simulink model "RadarSimulinkProjectRev011"  (R2024a)
settings: Solver=VariableStepAuto  StartTime=0.0  StopTime=0.0125*2  RelTol=1e-3
values from neighbouring files (symbols this model uses):
  AngleTime = SweepTime/10    (= 10000)    [InitializationOfVariablesRev000.m]    (also in InitializationOfVariablesRev001.m; InitializationOfVariablesRev002.m = 2000; InitializationOfVariablesRev003.m = 20000; InitializationOfVariablesRev004.m = 2097152)
  ASR_LUT = Rsamp    [InitializationOfVariablesRev003.m]    (also in InitializationOfVariablesRev004.m = round((R*2*SystemFs)/c); InitializationOfVariablesRev005.m = round((R*2*SystemFs)/c))
  Btn_Debounce = 20000    [InitializationOfVariablesRev003.m]    (also in InitializationOfVariablesRev004.m; InitializationOfVariablesRev005.m)
  ChirpNc = 128    [InitializationOfVariablesRev004.m]    (also in InitializationOfVariablesRev005.m)
  ChirpSizeLength = length(FCW)    [InitializationOfVariablesRev004.m]    (also in InitializationOfVariablesRev005.m = 16384)
  DeciFactor = 8    [InitializationOfVariablesRev005.m]
  FCW = [FCW_p1, FCW_p2]    [InitializationOfVariablesRev002.m]    (also in InitializationOfVariablesRev003.m; InitializationOfVariablesRev004.m = interp1(1:length(FCW_base), FCW_base,      linspace(1, lengt; InitializationOfVariablesRev005.m = f / SystemFs)
  RXFFTLength = 4096    [InitializationOfVariablesRev003.m]    (also in InitializationOfVariablesRev004.m = 1024; InitializationOfVariablesRev005.m = 2048)
  SweepTime = 100000    [InitializationOfVariablesRev000.m]    (also in InitializationOfVariablesRev001.m; InitializationOfVariablesRev002.m = 20000; InitializationOfVariablesRev003.m = 200000; InitializationOfVariablesRev004.m = 23068672)
undefined symbols (not defined in the file or in its folder): SignalGenerationForAnalysis, Subsystem, xc7a200tfbg676
libraries: hdlBasic x453, hdlUtilities x11, hdlDSPIP x11, vmcUtilities x1
(part 1 of 5)
settings Model: Creator=Cube II  LastModifiedBy=Cube II
settings ModelReferenceCC: UpdateModelReferenceTargets=IfOutOfDate

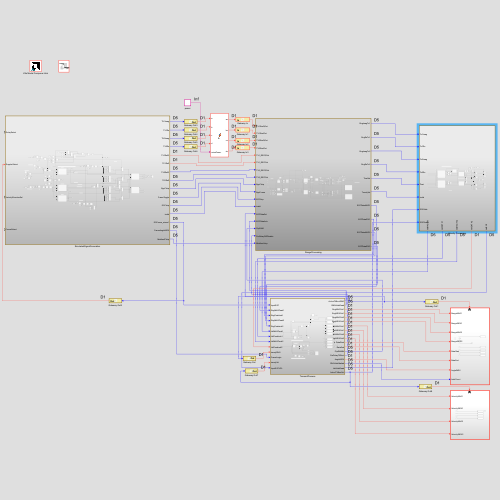
[thumbnail: Simulink's stored preview of the top-level diagram]
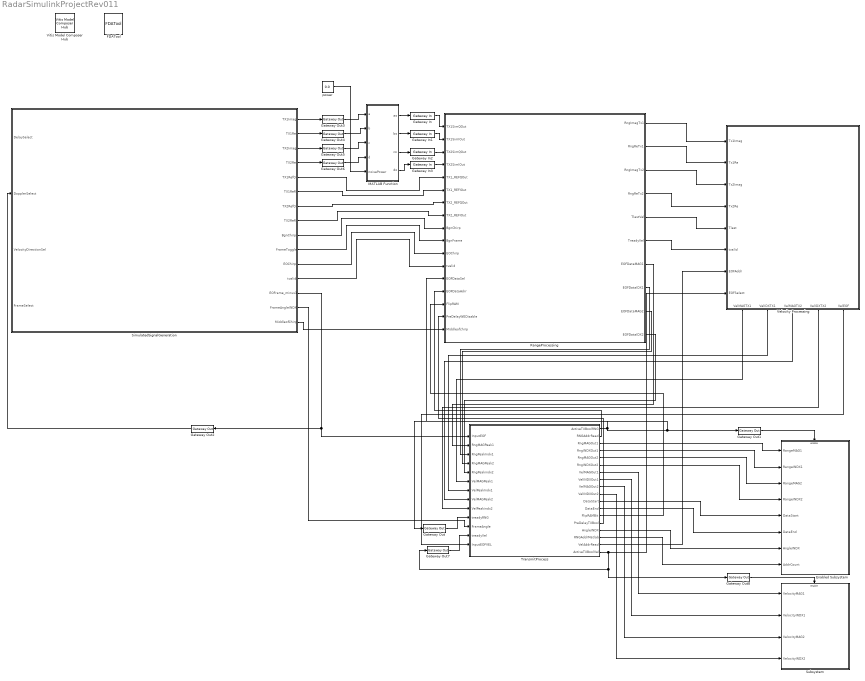
== system RadarSimulinkProjectRev011 ==
  Enabled Subsystem : Subsystem  TreatAsAtomicUnit=on
  FDATool : hdlUtilities/FDATool  block_type=fdatool
      settings: infoedit=FDATool
  Gateway In{,1..3} (4 alike) : hdlBasic/Gateway In  gui_display_data_type=Fixed-point  arith_type=Signed (2's comp)  n_bits=16  bin_pt=14  preci_type=Single  exp_width=8  frac_width=24  rows=1  columns=1  quantization="Round  (unbiased: +/- Inf)"  overflow=Saturate  period=P1  UseAsADC=off  ADCChannel='1'  interface=None  automatic_assignment=on  address_offset=hex2dec('00')  intf_name=''  intf_description=''  default_value=0  timing_constraint=None  locs_specified=off  LOCs={}  io_standard={}  inherit_from_input=off  hdl_port=on  XmcBlockStatus=1  maskContainerNames=group4  block_type=gatewayin  block_config=sysgen:gateway_in_config  block_width_w=590  block_height_w=620  block_width=640  block_height=850
  Gateway Out{,1..8} (9 alike) : hdlBasic/Gateway Out  inherit_from_input=off  bool_to_boolean=off  hdl_port=on  rows=1  columns=1  UseAsDAC=off  DACChannel='1'  interface=None  automatic_assignment=on  address_offset=hex2dec('00')  intf_name=''  intf_description=''  timing_constraint=None  locs_specified=off  LOCs={}  io_standard={}  XmcBlockStatus=1  maskContainerNames=group4  block_type=gatewayout  block_config=sysgen:gateway_out_config  block_width_w=590  block_height_w=620  block_width=620  block_height=750
  MATLAB Function : MATLAB Function  TreatAsAtomicUnit=on
  RangeProcessing : Subsystem
  SimulatedSignalGeneration : Subsystem  SystemSampleTime=1/200e6
  Subsystem : Subsystem
  TransmitProcess : Subsystem
  Velocity Processing : Subsystem
      settings: PortSchema="{\"entries\":[{\"content\":{\"sides\":[{\"content\":{\"connectorIds\":[\"In1\",\"In2\",\"In3\",\"In4\",\"In5\",\"In6\",\"In7\",\"In8\"]},\"type\":\"ConnectorPlacement.EquallySpacedRectSide\",\"uuid\":\"28660edc-4300-4d13-b5c7-cb230341ceef\"},{\"content\":{\"side\":\"RIGHT\"},\"type\":\"ConnectorPlacement.EquallySpacedRectSide\",\"uuid\":\"0aea0b64-dbd9-49d9-980c-6712e9fa4544\"},{\"content\":{\"side\":\"TOP\"},\"type\":\"ConnectorPlacement.EquallySpacedRectSide\",\"uuid\":\"4015706e-c6eb-4ca9-b4bb-31c510b09214\"},{\"content\":{\"connectorIds\":[\"Out1\",\"Out2\",\"Out3\",\"Out4\",\"Out5\"],\"side\":\"BOTTOM\"},\"type\":\"ConnectorPlacement.EquallySpacedRectSide\",\"uuid\":\"e3ca7ed1-345c-4783-9732-f7a0ff2c5995\"}]},\"type\":\"ConnectorPlacement.EquallySpacedConnector\",\"uuid\":\"ab051aed-e004-4640-a7d2-fe89028938d7\"}],\"packageUris\":[\"http://schema.mathworks.com/mf0/Connector/R2020b\"],\"version\":\"1.0\"}"
  Vitis Model Composer Hub : vmcUtilities/Vitis Model Composer Hub  Tag=genX  CodeGeneration=off  SubsystemName=RangeProcessing  BlockHierPath=SignalGenerationForAnalysis/Subsystem  CompilationType=HDLCompilation  SubsystemType=HDLNode  ExportTypeV2=IP Catalog  StartColumn=1  NumberOfColumns=1  TargetDirectory=./netlist  exportDesign=off  analyzeDesign=on  validateDesignOnHw=off  ExportType=AI Engines  IpVendor=xilinx.com  IpLibrary=hls  IpVersion=1.0  IpHWLanguage=Verilog  AieCompilerOptions={}  AieSimulatorOptions={}  CreateTestbench=on  TestbenchStackSize=10  RunRtlSim=off  RunCSim=off  RunAieSim=off  AieSimTimeout=50000  RunAieSimProfiling=off  LaunchVitisAnalyzer=off  PlotOutput=off  RunX86Sim=off  X86SimTimeout=10  GenHwImage=off  GenLibadfXo=on  GenHwValidationCode=off  PlatformType=Not Specified  HwSystemType=Baremetal  HwValidationTarget=hw  ProjDevice=Artix-7 AC701 Evaluation Platform (xc7a200tfbg676-2)  ProjDevicePart=xc7a200tfbg676-2  AIEType=None  SamplePeriod=-1  ClockFrequency=200  DataPathParallelism=1  xilinxfamily=artix7  part=xc7a200t  speed=-2  package=fbg676  directory=./netlist\ip\RangeProcessing\src  testbench=off  incr_netlist=off  synthesis_tool=Vivado  clock_wrapper=Clock Enables  dbl_ovrd=According to Block Masks  dcm_input_clock_period=10  sysclk_period=6.25  simulink_period=1/192e6  eval_field=0  IPInfoJsonString="{\"DUTSubsystemName\":\"Subsystem\",\"HDLSubsystem\":{\"SubsystemName\":\"Subsystem\",\"IPName\":\"Subsystem\",\"IPLibrary\":\"VMC\",\"IPVendor\":\"User Company\",\"IPVersion\":\"1.0\",\"TargetDirectory\":\"./netlist\",\"SubsystemDir\":\"./netlist\\\\ip\\\\Subsystem\",\"FreqHz\":\"200000000\"},\"SubsystemTag\":\"HDLNode\"}"  LogFileName=S:\RadarProjectSimulink\netlist\model_composer.log  NThreads=4  IPConfigFile=C:\Users\Cube II\AppData\Local\Temp\vmctmp-5941030035629153029\SignalGenerationForAnalysis_ipconfig.json
  power : Constant  Value=0.0
  wires:
  SimulatedSignalGeneration/3(TX2Imag) -> Gateway Out5/1
  SimulatedSignalGeneration/7(TX2RefQ) -> RangeProcessing/7(TX2_REFQOut)
  SimulatedSignalGeneration/8(TX2RefI) -> RangeProcessing/8(TX2_REFIOut)
  SimulatedSignalGeneration/10(FrameToggle) -> RangeProcessing/10(BgnFrame)
  SimulatedSignalGeneration/9(BgnChirp) -> RangeProcessing/9(BgnChirp)
  SimulatedSignalGeneration/2(TX1Re) -> Gateway Out4/1
  SimulatedSignalGeneration/1(TX1Imag) -> Gateway Out3/1
  SimulatedSignalGeneration/6(TX1RefI) -> RangeProcessing/6(TX1_REFIOut)
  SimulatedSignalGeneration/5(TX1RefQ) -> RangeProcessing/5(TX1_REFQOut)
  SimulatedSignalGeneration/11(EOChirp) -> RangeProcessing/11(EOChirp)
  SimulatedSignalGeneration/12(tvalid) -> RangeProcessing/12(tvalid)
  RangeProcessing/1(RngImagTx1) -> Velocity Processing/1(Tx1Imag)
  RangeProcessing/2(RngReTx1) -> Velocity Processing/2(Tx1Re)
  RangeProcessing/4(RngReTx2) -> Velocity Processing/4(Tx2Re)
  RangeProcessing/3(RngImagTx2) -> Velocity Processing/3(Tx2Imag)
  RangeProcessing/5(TlastVel) -> Velocity Processing/5(Tlast)
  RangeProcessing/6(TreadyVel) -> Velocity Processing/6(tvalid)
  SimulatedSignalGeneration/13(EOFrame_minus1) -> TransmitProcess/1(InputEOF), Gateway Out2/1
  TransmitProcess/1(ActiveTXBoolRNG) -> Gateway Out1/1, Gateway Out/1, RangeProcessing/13(EOFDataSel)
  TransmitProcess/2(RNGAddrRead) -> RangeProcessing/14(EOFDataAdrr)
  RangeProcessing/7(EOFDataMAG1) -> TransmitProcess/2(RngMAGPeak1)
  RangeProcessing/8(EOFDataIDX1) -> TransmitProcess/3(RngPeakIndx1)
  RangeProcessing/9(EOFDataMAG2) -> TransmitProcess/4(RngMAGPeak2)
  RangeProcessing/10(EOFDataIDX2) -> TransmitProcess/5(RngPeakindx2)
  Velocity Processing/1(VelMAGTX1) -> TransmitProcess/6(VelMAGPeak1)
  Velocity Processing/2(VelIDXTX1) -> TransmitProcess/7(VelPeakIndx1)
  Velocity Processing/3(VelMAGTX2) -> TransmitProcess/8(VelMAGPeak2)
  Velocity Processing/4(VelIDXTX2) -> TransmitProcess/9(VelPeakindx2)
  Gateway Out/1 -> TransmitProcess/10(treadyRNG)
  TransmitProcess/13(FlipRAMBit) -> RangeProcessing/15(FlipRAM)
  TransmitProcess/14(PreDelayTXBool) -> RangeProcessing/16(PreDelayWEDisable)
  TransmitProcess/3(RngMAGOut1) -> Enabled Subsystem/1(RangeMAG1)
  TransmitProcess/4(RngINDXOut1) -> Enabled Subsystem/2(RangeINDX1)
  TransmitProcess/5(RngMAGOut2) -> Enabled Subsystem/3(RangeMAG2)
  TransmitProcess/6(RngINDXOut2) -> Enabled Subsystem/4(RangeINDX2)
  TransmitProcess/10(VelINDXOut2) -> Subsystem/4(VelocityINDX2)
  TransmitProcess/11(DataStart) -> Enabled Subsystem/5(DataStart)
  TransmitProcess/12(DataEnd) -> Enabled Subsystem/6(DataEnd)
  Gateway Out1/1 -> Enabled Subsystem/Enable
  SimulatedSignalGeneration/14(FrameAngleINDX) -> TransmitProcess/11(FrameAngle)
  TransmitProcess/15(AngleINDX) -> Enabled Subsystem/7(AngleINDX)
  TransmitProcess/16(RNGAddrMatlab) -> Enabled Subsystem/8(AddrCount)
  Gateway Out2/1 -> SimulatedSignalGeneration/2(DopplerSelect)
  MATLAB Function/1(ao) -> Gateway In/1
  Gateway Out3/1 -> MATLAB Function/1(a)
  Gateway In/1 -> RangeProcessing/1(TX1SimQOut)
  power/1 -> MATLAB Function/5(noisePower)
  Gateway In1/1 -> RangeProcessing/2(TX1SimIOut)
  Gateway Out4/1 -> MATLAB Function/2(b)
  MATLAB Function/2(bo) -> Gateway In1/1
  Gateway In2/1 -> RangeProcessing/3(TX2SimQOut)
  Gateway In3/1 -> RangeProcessing/4(TX2SimIOut)
  SimulatedSignalGeneration/4(TX2Re) -> Gateway Out6/1
  Gateway Out5/1 -> MATLAB Function/3(c)
  Gateway Out6/1 -> MATLAB Function/4(d)
  MATLAB Function/3(co) -> Gateway In2/1
  MATLAB Function/4(do) -> Gateway In3/1
  SimulatedSignalGeneration/15(MiddleofChirp) -> RangeProcessing/17(Middleofchirp)
  TransmitProcess/17(VelAddrRead) -> Velocity Processing/7(EOFAddr)
  TransmitProcess/18(ActiveTXBoolVel) -> Gateway Out8/1, Gateway Out7/1, Velocity Processing/8(EOFSelect)
  TransmitProcess/9(VelMAGOut2) -> Subsystem/3(VelocityMAG2)
  TransmitProcess/8(VelINDXOut1) -> Subsystem/2(VelocityINDX1)
  TransmitProcess/7(VelMAGOut1) -> Subsystem/1(VelocityMAG1)
  Gateway Out7/1 -> TransmitProcess/12(treadyVel)
  Gateway Out8/1 -> Subsystem/Enable
  Velocity Processing/5(VelEOF) -> TransmitProcess/13(InputEOFVEL)

== system RadarSimulinkProjectRev011/Enabled Subsystem ==
  RangeMAG1 : Inport
  RangeINDX1 : Inport  Port=2
  RangeMAG2 : Inport  Port=3
  RangeINDX2 : Inport  Port=4
  DataStart : Inport  Port=5
  DataEnd : Inport  Port=6
  AngleINDX : Inport  Port=7
  AddrCount : Inport  Port=8
  Enable : EnablePort
  Terminator : Terminator
  To Workspace : ToWorkspace  VariableName=RangeMAG1  SampleTime=-1
      settings: Save2DSignal=2-D array (concatenate along first dimension)
  To Workspace1 : ToWorkspace  VariableName=RangeINDX1  SampleTime=-1
      settings: Save2DSignal=2-D array (concatenate along first dimension)
  To Workspace2 : ToWorkspace  VariableName=RangeMAG2  SampleTime=-1
      settings: Save2DSignal=2-D array (concatenate along first dimension)
  To Workspace3 : ToWorkspace  VariableName=RangeINDX2  SampleTime=-1
      settings: Save2DSignal=2-D array (concatenate along first dimension)
  To Workspace8 : ToWorkspace  VariableName=FrameNum  SampleTime=-1
      settings: Save2DSignal=2-D array (concatenate along first dimension)
  wires:
  DataStart/1 -> Terminator/1
  RangeMAG2/1 -> To Workspace2/1
  RangeINDX2/1 -> To Workspace3/1
  AngleINDX/1 -> To Workspace8/1
  RangeMAG1/1 -> To Workspace/1
  RangeINDX1/1 -> To Workspace1/1

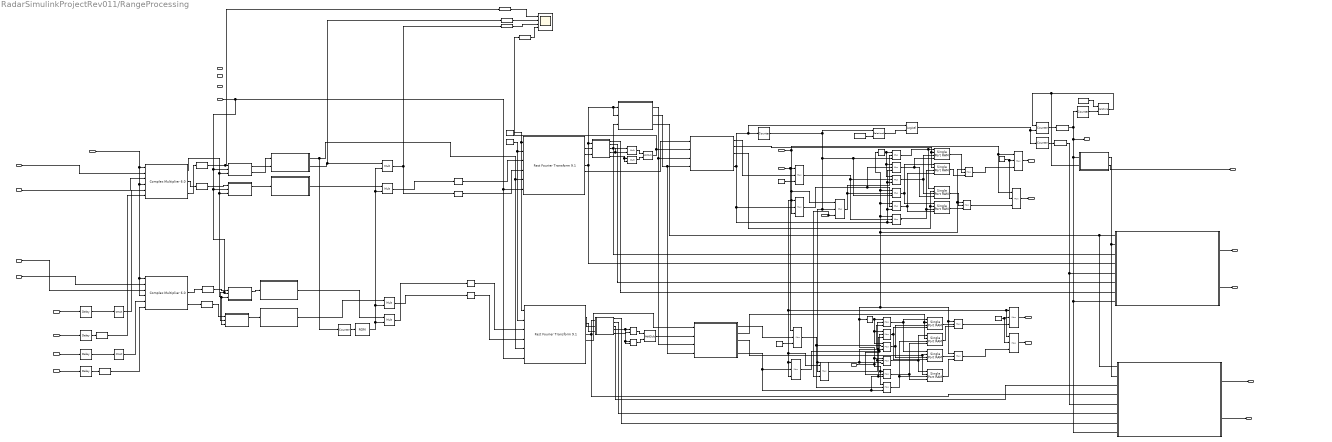
== system RadarSimulinkProjectRev011/RangeProcessing ==
  note: Based on results only 36 are completed for 0.0116 second time
      | 0.0464s required for 1 frame, so 1.02s, for 1 sweep, not counting for doppler fft time
  note: There should be only 128 tlasts over 10ms period
  note: Low Pass Fc=500kHz
  note: Tready will last until end of all samples, use for Doppler FFT
  note: These blocks are still needed for transmitting the range
  note: Will be 1 at PreDelay of EOF process, and 0 at end
      | 0 = pass through, 1 = STOP writting.
  note: Will switch to different RAM for doing the read operations, but delay not accounted
      | for the 50,000 sample delay for doppler FFT. Need to switch off WE and hold.
  note: Describes what chirp we are on, it's enable will trigger at the end of each FFT
  note: All Delays for after base Sig has been emitted
      | DDS (1) + CompMult (50) = (51)
  note: Delays per sample:
      | -Before Emittance (1)
      | -Simulated Signal (50)
      | -Recv Mixer (50)
      | -Windowing (3)
  note: TX1SimIOut
  note: TX1SimQOut
  note: TX2SimIOut
  note: TX2SimQOut
  note: TX1_REFIOut
  note: TX1_REFQOut
  note: TX2_REFIOut
  note: TX2_REFQOut
  note: Dechirp (mix with reference)
  note: WindowingFunction
  note: Windowing Multiplication
  note: For Syncronization: All references to frame and chirp switching need to be delayed only by the amount of delay between when it is called to toggle, and when it leaves the radar system.
      |
      | For any delay occuring within the simulation part after, this must be accounted for in the addressable shift register (delay) which simulates range delay. This delay has nothing to do with determinng when a chirp or frame has started/ended. The minimum delay, if not 0, will need to be acounted for.
      |
      | For any delay after reception, such as windowing or multiplication, this delay is relevant to anything that has to do with the processes that depend on knowing when a frame or chirp has started/ended. Since it should only start sampling once a signal theoretically should have arrived from 0 meters (no sim delay)
  note: All Delays After Dechirp
      | Delay = (101)
  note: Delay, accounting for sample missmatch
      | Delay = (104 + 139) = (243)
  note: Signal rate =12MHz
      | Sampling rate = 192MHz
  TX1SimQOut : Inport
  TX1SimIOut : Inport  Port=2
  TX2SimQOut : Inport  Port=3
  TX2SimIOut : Inport  Port=4
  TX1_REFQOut : Inport  Port=5
  TX1_REFIOut : Inport  Port=6
  TX2_REFQOut : Inport  Port=7
  TX2_REFIOut : Inport  Port=8
  BgnChirp : Inport  Port=9
  BgnFrame : Inport  Port=10
  EOChirp : Inport  Port=11
  tvalid : Inport  Port=12
  EOFDataSel : Inport  Port=13
  EOFDataAdrr : Inport  Port=14
  FlipRAM : Inport  Port=15
  PreDelayWEDisable : Inport  Port=16
  Middleofchirp : Inport  Port=17
  ADDRSwitch{,1..3} (4 alike) : hdlBasic/Mux  inputs=2  en=off  latency=0  precision=Full  arith_type=Unsigned  n_bits=16  bin_pt=14  quantization=Truncate  overflow=Wrap  XmcBlockStatus=1  maskContainerNames=tabcontainer1  block_type=mux  block_config=sysgen:Mux_config
  AddSub : hdlBasic/AddSub  mode=Addition  use_carryin=off  use_carryout=off  en=off  latency=0  precision=Full  arith_type=Unsigned  n_bits=16  bin_pt=14  quantization=Truncate  overflow=Wrap  use_behavioral_HDL=off  hw_selection=Fabric  pipelined=off  XmcBlockStatus=1  maskContainerNames=tabcontainer1  block_type=addsub  block_config=sysgen:Addsub_config
  AddSub1 : hdlBasic/AddSub  mode=Addition  use_carryin=off  use_carryout=off  en=off  latency=0  precision=Full  arith_type=Unsigned  n_bits=16  bin_pt=14  quantization=Truncate  overflow=Wrap  use_behavioral_HDL=off  hw_selection=Fabric  pipelined=off  XmcBlockStatus=1  maskContainerNames=tabcontainer1  block_type=addsub  block_config=sysgen:Addsub_config
  AddrCountPerChirp : hdlBasic/Counter  cnt_type=Count limited  cnt_to=ChirpNc-1  operation=Up  start_count=0  cnt_by_val=1  arith_type=Unsigned  n_bits=7  bin_pt=0  load_pin=off  rst=off  en=on  explicit_period=Explicit  period=P1  use_behavioral_HDL=off  implementation=Fabric  XmcBlockStatus=1  maskContainerNames=group1  block_type=counter  block_config=sysgen:Counter_config  block_width=531  block_height=1023
  CMult : hdlBasic/CMult  const=-1  gui_display_data_type=Fixed-point  const_n_bits=1  const_bin_pt=0  float_type=Single  exp_bits=8  fraction_bits=24  en=off  latency=0  precision=Full  arith_type="Signed  (2's comp)"  n_bits=16  bin_pt=14  quantization=Truncate  overflow=Wrap  use_behavioral_HDL=off  mem_type=Distributed RAM  pipeline=off  XmcBlockStatus=1  maskContainerNames=tabcontainer1  block_type=cmult  block_config=sysgen:CMult_config
      settings: infoedit=[]
  CMult1 : hdlBasic/CMult  const=-1  gui_display_data_type=Fixed-point  const_n_bits=1  const_bin_pt=0  float_type=Single  exp_bits=8  fraction_bits=24  en=off  latency=0  precision=Full  arith_type="Signed  (2's comp)"  n_bits=16  bin_pt=14  quantization=Truncate  overflow=Wrap  use_behavioral_HDL=off  mem_type=Distributed RAM  pipeline=off  XmcBlockStatus=1  maskContainerNames=tabcontainer1  block_type=cmult  block_config=sysgen:CMult_config
      settings: infoedit=[]
  ChirpSamples : hdlBasic/Constant  const=ChirpNc*RXFFTLength-1  gui_display_data_type=Fixed-point  arith_type=Unsigned  n_bits=32  bin_pt=0  preci_type=Single  exp_width=8  frac_width=24  explicit_period=on  period=P2  XmcBlockStatus=1  maskContainerNames=tabcontainer1  block_type=constant  block_config=sysgen:Constant_config
  Complex Multiplier 6.1 : hdlDSPIP/Complex Multiplier 6.0   datatype=integer  hasatlast=off  hasatuser=off  atuserwidth=1  hasbtlast=off  hasbtuser=off  btuserwidth=1  multtype=Use_Mults  optimizegoal=Resources  flowcontrol=NonBlocking  outputwidth=34  roundmode=Truncate  hasctrltlast=off  hasctrltuser=off  ctrltuserwidth=1  outtlastbehv=Null  latencyconfig=Automatic  minimumlatency=37  aclken=off  aresetn=off  trim_axipin_name=on  simulation_type=hybrid_sim  simulation_model=sysgen:cmpy_v6_0  data_path_portlist={ 's_axis_a_tdata_real', 's_axis_a_tdata_imag', 's_axis_b_tdata_real', 's_axis_b_tdata_imag', 's_axis_ctrl_tdata_rounding_bit', 'm_axis_dout_tdata_real', 'm_axis_dout_tdata_imag' }  aportwidth=63  bportwidth=63  ip_name=Complex Multiplier  ip_version=6.0  dsptool_ready=true  ipcore_usecache=true  ipcore_useipmodelcache=true  ipcore_verbose=false  ipcore_latency_parameter='minimumlatency'  wrapper_available=true  port_translation_map={ 'aclken' => 'en', 'aresetn' => 'rst'}  XmcBlockStatus=1  maskContainerNames=tabcontainer1  block_type=cmpy_v6_0  block_config=sysgen:rodinimport_config
  Complex Multiplier 6.2 : hdlDSPIP/Complex Multiplier 6.0   datatype=integer  hasatlast=off  hasatuser=off  atuserwidth=1  hasbtlast=off  hasbtuser=off  btuserwidth=1  multtype=Use_Mults  optimizegoal=Resources  flowcontrol=NonBlocking  outputwidth=34  roundmode=Truncate  hasctrltlast=off  hasctrltuser=off  ctrltuserwidth=1  outtlastbehv=Null  latencyconfig=Automatic  minimumlatency=37  aclken=off  aresetn=off  trim_axipin_name=on  simulation_type=hybrid_sim  simulation_model=sysgen:cmpy_v6_0  data_path_portlist={ 's_axis_a_tdata_real', 's_axis_a_tdata_imag', 's_axis_b_tdata_real', 's_axis_b_tdata_imag', 's_axis_ctrl_tdata_rounding_bit', 'm_axis_dout_tdata_real', 'm_axis_dout_tdata_imag' }  aportwidth=63  bportwidth=63  ip_name=Complex Multiplier  ip_version=6.0  dsptool_ready=true  ipcore_usecache=true  ipcore_useipmodelcache=true  ipcore_verbose=false  ipcore_latency_parameter='minimumlatency'  wrapper_available=true  port_translation_map={ 'aclken' => 'en', 'aresetn' => 'rst'}  XmcBlockStatus=1  maskContainerNames=tabcontainer1  block_type=cmpy_v6_0  block_config=sysgen:rodinimport_config
  Constant4 : hdlBasic/Constant  const=0  gui_display_data_type=Boolean  arith_type=Boolean  n_bits=16  bin_pt=15  preci_type=Single  exp_width=8  frac_width=24  explicit_period=on  period=P2  XmcBlockStatus=1  maskContainerNames=tabcontainer1  block_type=constant  block_config=sysgen:Constant_config
  Constant5 : hdlBasic/Constant  const=0  gui_display_data_type=Boolean  arith_type=Boolean  n_bits=16  bin_pt=15  preci_type=Single  exp_width=8  frac_width=24  explicit_period=on  period=P2  XmcBlockStatus=1  maskContainerNames=tabcontainer1  block_type=constant  block_config=sysgen:Constant_config
  Constant6 : hdlBasic/Constant  const=0  gui_display_data_type=Fixed-point  arith_type=Signed (2's comp)  n_bits=16  bin_pt=15  preci_type=Single  exp_width=8  frac_width=24  explicit_period=on  period=P2  XmcBlockStatus=1  maskContainerNames=tabcontainer1  block_type=constant  block_config=sysgen:Constant_config
  Constant7 : hdlBasic/Constant  const=0  gui_display_data_type=Fixed-point  arith_type=Signed (2's comp)  n_bits=16  bin_pt=15  preci_type=Single  exp_width=8  frac_width=24  explicit_period=on  period=P2  XmcBlockStatus=1  maskContainerNames=tabcontainer1  block_type=constant  block_config=sysgen:Constant_config
  Convert : hdlBasic/Convert  gui_display_data_type=Fixed-point  arith_type=Signed (2's comp)  n_bits=17  bin_pt=15  float_type=Single  exp_bits=8  fraction_bits=24  quantization=Truncate  overflow=Wrap  en=off  latency=0  pipeline=off  XmcBlockStatus=1  maskContainerNames=group2  block_type=convert  block_config=sysgen:Convert_config  block_width=595  block_height=885
  Convert1 : hdlBasic/Convert  gui_display_data_type=Fixed-point  arith_type=Signed (2's comp)  n_bits=17  bin_pt=15  float_type=Single  exp_bits=8  fraction_bits=24  quantization=Truncate  overflow=Wrap  en=off  latency=0  pipeline=off  XmcBlockStatus=1  maskContainerNames=group2  block_type=convert  block_config=sysgen:Convert_config  block_width=595  block_height=885
  Convert{2..5} (4 alike) : hdlBasic/Convert  gui_display_data_type=Fixed-point  arith_type=Signed (2's comp)  n_bits=16  bin_pt=15  float_type=Single  exp_bits=8  fraction_bits=24  quantization="Round  (unbiased: +/- Inf)"  overflow=Saturate  en=off  latency=0  pipeline=off  XmcBlockStatus=1  maskContainerNames=group2  block_type=convert  block_config=sysgen:Convert_config  block_width=595  block_height=885
  Convert{6..9} (4 alike) : hdlBasic/Convert  gui_display_data_type=Fixed-point  arith_type=Signed (2's comp)  n_bits=24  bin_pt=10  float_type=Single  exp_bits=8  fraction_bits=24  quantization="Round  (unbiased: Even Values)"  overflow=Saturate  en=off  latency=0  pipeline=off  XmcBlockStatus=1  maskContainerNames=group2  block_type=convert  block_config=sysgen:Convert_config  block_width=595  block_height=885
  Counter2 : hdlBasic/Counter  cnt_type=Count limited  cnt_to=(ChirpNc*RXFFTLength)-1  operation=Up  start_count=0  cnt_by_val=1  arith_type=Unsigned  n_bits=18  bin_pt=0  load_pin=off  rst=off  en=on  explicit_period=Explicit  period=P1  use_behavioral_HDL=off  implementation=Fabric  XmcBlockStatus=1  maskContainerNames=group1  block_type=counter  block_config=sysgen:Counter_config  block_width=531  block_height=1023
  DC Removal : Subsystem
  DC Removal1 : Subsystem
  DC Removal2 : Subsystem
  DC Removal3 : Subsystem
  Delay{,1..3} (4 alike) : hdlBasic/Delay  rst=off  en=off  latency=6  reg_retiming=off  XmcBlockStatus=1  maskContainerNames=group1  block_type=delay  block_config=sysgen:Delay_config
  ENSwitch{,1..3} (4 alike) : hdlBasic/Mux  inputs=2  en=off  latency=0  precision=Full  arith_type=Unsigned  n_bits=16  bin_pt=14  quantization=Truncate  overflow=Wrap  XmcBlockStatus=1  maskContainerNames=tabcontainer1  block_type=mux  block_config=sysgen:Mux_config
  EOFRAADDR : hdlBasic/Mux  inputs=2  en=off  latency=0  precision=Full  arith_type=Unsigned  n_bits=16  bin_pt=14  quantization=Truncate  overflow=Wrap  XmcBlockStatus=1  maskContainerNames=tabcontainer1  block_type=mux  block_config=sysgen:Mux_config
  EOFRAADDR2 : hdlBasic/Mux  inputs=2  en=off  latency=0  precision=Full  arith_type=Unsigned  n_bits=16  bin_pt=14  quantization=Truncate  overflow=Wrap  XmcBlockStatus=1  maskContainerNames=tabcontainer1  block_type=mux  block_config=sysgen:Mux_config
  EOFRAMen1 : hdlBasic/Mux  inputs=2  en=off  latency=0  precision=Full  arith_type=Unsigned  n_bits=16  bin_pt=14  quantization=Truncate  overflow=Wrap  XmcBlockStatus=1  maskContainerNames=tabcontainer1  block_type=mux  block_config=sysgen:Mux_config
  EOFRAMen3 : hdlBasic/Mux  inputs=2  en=off  latency=0  precision=Full  arith_type=Unsigned  n_bits=16  bin_pt=14  quantization=Truncate  overflow=Wrap  XmcBlockStatus=1  maskContainerNames=tabcontainer1  block_type=mux  block_config=sysgen:Mux_config
  EOFRAMwe1 : hdlBasic/Mux  inputs=2  en=off  latency=0  precision=Full  arith_type=Unsigned  n_bits=16  bin_pt=14  quantization=Truncate  overflow=Wrap  XmcBlockStatus=1  maskContainerNames=tabcontainer1  block_type=mux  block_config=sysgen:Mux_config
  EOFRAMwe2 : hdlBasic/Mux  inputs=2  en=off  latency=0  precision=Full  arith_type=Unsigned  n_bits=16  bin_pt=14  quantization=Truncate  overflow=Wrap  XmcBlockStatus=1  maskContainerNames=tabcontainer1  block_type=mux  block_config=sysgen:Mux_config
  FFTResultRAMSystem : Subsystem
  FFTResultRAMSystem1 : Subsystem
  FFTSamplingRelation : hdlBasic/Relational  mode=a=b  op_type=Bool  en=off  latency=0  XmcBlockStatus=1  maskContainerNames=tabcontainer1  block_type=relational  block_config=sysgen:Relational_config
  FFTTracking : Subsystem
  FFT_C1 : hdlBasic/Constant  const=1.0  gui_display_data_type=Fixed-point  arith_type=Unsigned  n_bits=1  bin_pt=0  preci_type=Single  exp_width=8  frac_width=24  explicit_period=on  period=P2  XmcBlockStatus=1  maskContainerNames=tabcontainer1  block_type=constant  block_config=sysgen:Constant_config
  FFT_C2 : hdlBasic/Constant  const=1.0  gui_display_data_type=Boolean  arith_type=Boolean  n_bits=1  bin_pt=0  preci_type=Single  exp_width=8  frac_width=24  explicit_period=on  period=P2  XmcBlockStatus=1  maskContainerNames=tabcontainer1  block_type=constant  block_config=sysgen:Constant_config
  Fast Fourier Transform 9.1 : hdlDSPIP/Fast Fourier Transform 9.1   transform_length=16384  target_clock_frequency=192  target_data_throughput=50  implementation_options=pipelined_streaming_io  run_time_configurable_transform_length=off  enable_ssr=off  super_sample_rates=1  data_format=fixed_point  phase_factor_width=32  scaling_options=unscaled  rounding_modes=convergent_rounding  aclken=off  aresetn=off  output_ordering=natural_order  cyclic_prefix_insertion=off  throttle_scheme=realtime  xk_index=on  ovflo=off  trim_axipin_name=on  memory_options_data=block_ram  memory_options_phase_factors=block_ram  number_of_stages_using_block_ram_for_data_and_phase_factors=9  memory_options_reorder=block_ram  memory_options_hybrid=off  complex_mult_type=use_mults_resources  butterfly_type=use_xtremedsp_slices  simulation_type=hybrid_sim  simulation_model=sysgen:xfftv9_cmodel  data_path_portlist={ 's_axis_data_tdata', 'm_axis_data_tdata', 'm_axis_status_tdata', 'event_fft_overflow' }  channels=1  input_ordering=natural_order  input_width=16  ip_name=Fast Fourier Transform  ip_version=9.1  dsptool_ready=true  ipcore_usecache=true  ipcore_useipmodelcache=true  wrapper_available=true  port_translation_map={ 'aclken' => 'en', 'aresetn' => 'rst'}  XmcBlockStatus=1  maskContainerNames=tabcontainer1  block_type=xfft_v9_1  block_config=sysgen:rodinimport_config
  Fast Fourier Transform 9.2 : hdlDSPIP/Fast Fourier Transform 9.1   transform_length=16384  target_clock_frequency=192  target_data_throughput=50  implementation_options=pipelined_streaming_io  run_time_configurable_transform_length=off  enable_ssr=off  super_sample_rates=1  data_format=fixed_point  phase_factor_width=32  scaling_options=unscaled  rounding_modes=convergent_rounding  aclken=off  aresetn=off  output_ordering=natural_order  cyclic_prefix_insertion=off  throttle_scheme=realtime  xk_index=on  ovflo=off  trim_axipin_name=on  memory_options_data=block_ram  memory_options_phase_factors=block_ram  number_of_stages_using_block_ram_for_data_and_phase_factors=9  memory_options_reorder=block_ram  memory_options_hybrid=off  complex_mult_type=use_mults_resources  butterfly_type=use_xtremedsp_slices  simulation_type=hybrid_sim  simulation_model=sysgen:xfftv9_cmodel  data_path_portlist={ 's_axis_data_tdata', 'm_axis_data_tdata', 'm_axis_status_tdata', 'event_fft_overflow' }  channels=1  input_ordering=natural_order  input_width=16  ip_name=Fast Fourier Transform  ip_version=9.1  dsptool_ready=true  ipcore_usecache=true  ipcore_useipmodelcache=true  wrapper_available=true  port_translation_map={ 'aclken' => 'en', 'aresetn' => 'rst'}  XmcBlockStatus=1  maskContainerNames=tabcontainer1  block_type=xfft_v9_1  block_config=sysgen:rodinimport_config
  Gateway Out{9..12} (4 alike) : hdlBasic/Gateway Out  inherit_from_input=off  bool_to_boolean=off  hdl_port=on  rows=1  columns=1  UseAsDAC=off  DACChannel='1'  interface=None  automatic_assignment=on  address_offset=hex2dec('00')  intf_name=''  intf_description=''  timing_constraint=None  locs_specified=off  LOCs={}  io_standard={}  XmcBlockStatus=1  maskContainerNames=group4  block_type=gatewayout  block_config=sysgen:gateway_out_config  block_width_w=590  block_height_w=620  block_width=620  block_height=750
  INDXOutSwitch : hdlBasic/Mux  inputs=2  en=off  latency=0  precision=Full  arith_type=Unsigned  n_bits=16  bin_pt=14  quantization=Truncate  overflow=Wrap  XmcBlockStatus=1  maskContainerNames=tabcontainer1  block_type=mux  block_config=sysgen:Mux_config
  INDXOutSwitch1 : hdlBasic/Mux  inputs=2  en=off  latency=0  precision=Full  arith_type=Unsigned  n_bits=16  bin_pt=14  quantization=Truncate  overflow=Wrap  XmcBlockStatus=1  maskContainerNames=tabcontainer1  block_type=mux  block_config=sysgen:Mux_config
  Inverter : hdlBasic/Inverter  en=off  latency=0  XmcBlockStatus=1  maskContainerNames=group2  block_type=inv  block_config=sysgen:Inverter_config
  Inverter1 : hdlBasic/Inverter  en=off  latency=0  XmcBlockStatus=1  maskContainerNames=group2  block_type=inv  block_config=sysgen:Inverter_config
  LastChirp : hdlBasic/Constant  const=127  gui_display_data_type=Fixed-point  arith_type=Unsigned  n_bits=7  bin_pt=0  preci_type=Single  exp_width=8  frac_width=24  explicit_period=on  period=P2  XmcBlockStatus=1  maskContainerNames=tabcontainer1  block_type=constant  block_config=sysgen:Constant_config
  Logical : hdlBasic/Logical  logical_function=AND  inputs=2  en=off  latency=0  precision=Full  arith_type=Unsigned  n_bits=16  bin_pt=0  align_bp=on  overflow=[]  quantization=[]  XmcBlockStatus=1  maskContainerNames=tabcontainer1  block_type=logical  block_config=sysgen:Logical_config
  MAGOutSwitch : hdlBasic/Mux  inputs=2  en=off  latency=0  precision=Full  arith_type=Unsigned  n_bits=16  bin_pt=14  quantization=Truncate  overflow=Wrap  XmcBlockStatus=1  maskContainerNames=tabcontainer1  block_type=mux  block_config=sysgen:Mux_config
  MAGOutSwitch1 : hdlBasic/Mux  inputs=2  en=off  latency=0  precision=Full  arith_type=Unsigned  n_bits=16  bin_pt=14  quantization=Truncate  overflow=Wrap  XmcBlockStatus=1  maskContainerNames=tabcontainer1  block_type=mux  block_config=sysgen:Mux_config
  ManualDownsample1 : Subsystem
  ManualDownsample2 : Subsystem
  Mult{4..7} (4 alike) : hdlBasic/Mult  precision=Full  arith_type="Signed  (2's comp)"  n_bits=16  bin_pt=14  quantization=Truncate  overflow=Wrap  en=off  latency=3  opt_float=off  fp_mult_usage=No Usage  use_behavioral_HDL=off  opt=Speed  use_embedded=on  optimum_pipeline=off  pipeline=on  use_rpm=on  placement_style=Triangular  XmcBlockStatus=1  maskContainerNames=group1  block_type=mult  block_config=sysgen:Mult_config  block_width=598  block_height=876
  Mux{16..19} (4 alike) : hdlBasic/Mux  inputs=2  en=off  latency=0  precision=Full  arith_type=Unsigned  n_bits=16  bin_pt=14  quantization=Truncate  overflow=Wrap  XmcBlockStatus=1  maskContainerNames=tabcontainer1  block_type=mux  block_config=sysgen:Mux_config
  Peak Detection1 : Subsystem
  Peak Detection2 : Subsystem
  PeakAmp RAM{1..4} (4 alike) : hdlBasic/Single Port RAM  depth=ChirpNc  initVector=0  distributed_mem=Block RAM  write_mode=Read After Write  rst=off  init_reg=0  en=on  optimize_latency=off  latency=1  optimize=Area  dbl_ovrd=off  simulation_type=fast_sim  XmcBlockStatus=1  maskContainerNames=tabcontainer1  block_type=spram  block_config=sysgen:SPRAM_config
  PeakIndx RAM{1..4} (4 alike) : hdlBasic/Single Port RAM  depth=ChirpNc  initVector=0  distributed_mem=Block RAM  write_mode=Read After Write  rst=off  init_reg=0  en=on  optimize_latency=off  latency=1  optimize=Area  dbl_ovrd=off  simulation_type=fast_sim  XmcBlockStatus=1  maskContainerNames=tabcontainer1  block_type=spram  block_config=sysgen:SPRAM_config
  ROM : hdlBasic/ROM  depth=ChirpSizeLength  initVector=WindowCoefficients  distributed_mem=Block RAM  rst=off  init_reg=0  en=off  latency=1  gui_display_data_type=Fixed-point  arith_type=Unsigned  n_bits=16  bin_pt=15  preci_type=Single  exp_width=8  frac_width=24  optimize=Area  use_rpm=on  simulation_type=fast_sim  XmcBlockStatus=1  maskContainerNames=tabcontainer1  block_type=sprom  block_config=sysgen:SPROM_config
  RX Lowpass Filter : Subsystem
  RX Lowpass Filter1 : Subsystem
  RX Lowpass Filter2 : Subsystem
  RX Lowpass Filter3 : Subsystem
  ReadENBool : hdlBasic/Convert  gui_display_data_type=Boolean  arith_type=Boolean  n_bits=16  bin_pt=14  float_type=Single  exp_bits=8  fraction_bits=24  quantization=Truncate  overflow=Wrap  en=off  latency=0  pipeline=off  XmcBlockStatus=1  maskContainerNames=group2  block_type=convert  block_config=sysgen:Convert_config  block_width=595  block_height=885
  ReadENBool1 : hdlBasic/Convert  gui_display_data_type=Boolean  arith_type=Boolean  n_bits=16  bin_pt=14  float_type=Single  exp_bits=8  fraction_bits=24  quantization=Truncate  overflow=Wrap  en=off  latency=0  pipeline=off  XmcBlockStatus=1  maskContainerNames=group2  block_type=convert  block_config=sysgen:Convert_config  block_width=595  block_height=885
  ReadENCounter : hdlBasic/Counter  cnt_type=Count limited  cnt_to=1  operation=Up  start_count=0  cnt_by_val=1  arith_type=Unsigned  n_bits=1  bin_pt=0  load_pin=off  rst=on  en=on  explicit_period=Explicit  period=P1  use_behavioral_HDL=off  implementation=Fabric  XmcBlockStatus=1  maskContainerNames=group1  block_type=counter  block_config=sysgen:Counter_config  block_width=531  block_height=1023
  ReadToggleBool : hdlBasic/Counter  cnt_type=Count limited  cnt_to=1  operation=Up  start_count=0  cnt_by_val=1  arith_type=Unsigned  n_bits=1  bin_pt=0  load_pin=off  rst=off  en=on  explicit_period=Explicit  period=P1  use_behavioral_HDL=off  implementation=Fabric  XmcBlockStatus=1  maskContainerNames=group1  block_type=counter  block_config=sysgen:Counter_config  block_width=531  block_height=1023
  Scope3 : Scope  NumInputPorts=4
  Subsystem : Subsystem
  TlastChirpRelation : hdlBasic/Relational  mode=a=b  op_type=Bool  en=off  latency=0  XmcBlockStatus=1  maskContainerNames=tabcontainer1  block_type=relational  block_config=sysgen:Relational_config
  WeSwitch{1..4} (4 alike) : hdlBasic/Mux  inputs=2  en=off  latency=0  precision=Full  arith_type=Unsigned  n_bits=16  bin_pt=14  quantization=Truncate  overflow=Wrap  XmcBlockStatus=1  maskContainerNames=tabcontainer1  block_type=mux  block_config=sysgen:Mux_config
  WinImag1 : hdlBasic/Mult  precision=Full  arith_type="Signed  (2's comp)"  n_bits=16  bin_pt=14  quantization=Truncate  overflow=Wrap  en=off  latency=0  opt_float=off  fp_mult_usage=No Usage  use_behavioral_HDL=off  opt=Speed  use_embedded=on  optimum_pipeline=off  pipeline=on  use_rpm=on  placement_style=Triangular  XmcBlockStatus=1  maskContainerNames=group1  block_type=mult  block_config=sysgen:Mult_config  block_width=598  block_height=876
  WinImag2 : hdlBasic/Mult  precision=Full  arith_type="Signed  (2's comp)"  n_bits=16  bin_pt=14  quantization=Truncate  overflow=Wrap  en=off  latency=0  opt_float=off  fp_mult_usage=No Usage  use_behavioral_HDL=off  opt=Speed  use_embedded=on  optimum_pipeline=off  pipeline=on  use_rpm=on  placement_style=Triangular  XmcBlockStatus=1  maskContainerNames=group1  block_type=mult  block_config=sysgen:Mult_config  block_width=598  block_height=876
  WinReal1 : hdlBasic/Mult  precision=Full  arith_type="Signed  (2's comp)"  n_bits=16  bin_pt=14  quantization=Truncate  overflow=Wrap  en=off  latency=0  opt_float=off  fp_mult_usage=No Usage  use_behavioral_HDL=off  opt=Speed  use_embedded=on  optimum_pipeline=off  pipeline=on  use_rpm=on  placement_style=Triangular  XmcBlockStatus=1  maskContainerNames=group1  block_type=mult  block_config=sysgen:Mult_config  block_width=598  block_height=876
  WinReal2 : hdlBasic/Mult  precision=Full  arith_type="Signed  (2's comp)"  n_bits=16  bin_pt=14  quantization=Truncate  overflow=Wrap  en=off  latency=0  opt_float=off  fp_mult_usage=No Usage  use_behavioral_HDL=off  opt=Speed  use_embedded=on  optimum_pipeline=off  pipeline=on  use_rpm=on  placement_style=Triangular  XmcBlockStatus=1  maskContainerNames=group1  block_type=mult  block_config=sysgen:Mult_config  block_width=598  block_height=876
  WindowPeriod : hdlBasic/Counter  cnt_type=Count limited  cnt_to=ChirpSizeLength-1  operation=Up  start_count=0  cnt_by_val=1  arith_type=Unsigned  n_bits=14  bin_pt=0  load_pin=off  rst=off  en=on  explicit_period=Explicit  period=P1  use_behavioral_HDL=off  implementation=Fabric  XmcBlockStatus=1  maskContainerNames=group1  block_type=counter  block_config=sysgen:Counter_config  block_width=531  block_height=1023
  RngImagTx1 : Outport
  RngReTx1 : Outport  Port=2
  RngImagTx2 : Outport  Port=3
  RngReTx2 : Outport  Port=4
  TlastVel : Outport  Port=5
  TreadyVel : Outport  Port=6
  EOFDataMAG1 : Outport  Port=7
  EOFDataIDX1 : Outport  Port=8
  EOFDataMAG2 : Outport  Port=9
  EOFDataIDX2 : Outport  Port=10
  wires:
  WindowPeriod/1 -> ROM/1
  FFT_C1/1 -> Fast Fourier Transform 9.1/1, Fast Fourier Transform 9.2/1
  CMult1/1 -> Complex Multiplier 6.2/5
  TX1_REFIOut/1 -> Delay1/1
  CMult/1 -> Complex Multiplier 6.1/5
  TX2_REFIOut/1 -> Delay3/1
  FFT_C2/1 -> Fast Fourier Transform 9.1/2, Fast Fourier Transform 9.2/2
  Fast Fourier Transform 9.1/7 -> Peak Detection2/1(Tlast)
  tvalid/1 -> Complex Multiplier 6.2/1, Complex Multiplier 6.2/4, Complex Multiplier 6.1/4, Complex Multiplier 6.1/1
  ManualDownsample2/1(IMG) -> FFTResultRAMSystem/7(DataIMG)
  ManualDownsample2/2(RE) -> FFTResultRAMSystem/6(DataRE)
  Mult6/1 -> AddSub1/2
  Mult7/1 -> AddSub1/1
  AddSub1/1 -> Peak Detection1/2(FFTInput)
  LastChirp/1 -> TlastChirpRelation/2
  Logical/1 -> ReadToggleBool/1, ReadENCounter/2  "TLast"
  TlastChirpRelation/1 -> Logical/2  "TLast"
  ReadENCounter/1 -> ReadENBool/1
  Counter2/1 -> FFTSamplingRelation/2
  ChirpSamples/1 -> FFTSamplingRelation/1
  FFTSamplingRelation/1 -> ReadENCounter/1, Subsystem/2(Reset)  "TLast"
  EOFRAMwe1/1 -> WeSwitch3/2, WeSwitch2/2
  EOFRAMen1/1 -> ENSwitch3/2, ENSwitch2/2
  Constant4/1 -> EOFRAMwe1/3
  EOFRAADDR2/1 -> ADDRSwitch3/2, ADDRSwitch2/2
  PeakAmp RAM2/1 -> MAGOutSwitch/2  "MAGPeak2"
  PeakIndx RAM2/1 -> INDXOutSwitch/2
  EOFDataAdrr/1 -> EOFRAADDR/3, EOFRAADDR2/3
  EOFRAADDR/1 -> ADDRSwitch1/2, ADDRSwitch/2
  AddrCountPerChirp/1 -> EOFRAADDR/2, ADDRSwitch1/3, ADDRSwitch/3, EOFRAADDR2/2, ADDRSwitch2/3, ADDRSwitch3/3, TlastChirpRelation/1
  EOFRAMen3/1 -> ENSwitch/2, ENSwitch1/2
  EOFRAMwe2/1 -> WeSwitch4/2, WeSwitch1/2
  Constant5/1 -> EOFRAMwe2/3
  INDXOutSwitch1/1 -> Mux17/3
  PeakIndx RAM1/1 -> INDXOutSwitch1/2  "PeakIndx1"
  MAGOutSwitch1/1 -> Mux16/3
  PeakAmp RAM1/1 -> MAGOutSwitch1/2  "MAGPeak1"
  Constant6/1 -> Mux17/2, Mux16/2
  Mux16/1 -> EOFDataMAG1/1
  Mux17/1 -> EOFDataIDX1/1
  INDXOutSwitch/1 -> Mux19/3
  EOFDataSel/1 -> EOFRAADDR2/1, EOFRAADDR/1, EOFRAMen3/3, EOFRAMen3/1, Mux19/1, Mux18/1, EOFRAMen1/3, EOFRAMen1/1, Mux16/1, Mux17/1
  Constant7/1 -> Mux18/2, Mux19/2
  MAGOutSwitch/1 -> Mux18/3
  Mux19/1 -> EOFDataIDX2/1
  Inverter/1 -> WeSwitch4/1, ENSwitch1/1, ADDRSwitch1/1
  Inverter1/1 -> WeSwitch3/1, ENSwitch3/1, ADDRSwitch3/1
  FlipRAM/1 -> WeSwitch1/1, ENSwitch/1, Inverter1/1, ADDRSwitch2/1, ENSwitch2/1, WeSwitch2/1, INDXOutSwitch1/1, MAGOutSwitch1/1, INDXOutSwitch/1, MAGOutSwitch/1, Inverter/1, ADDRSwitch/1
  ENSwitch/1 -> PeakIndx RAM3/4, PeakAmp RAM3/4
  WeSwitch1/1 -> PeakAmp RAM3/3, PeakIndx RAM3/3
  ADDRSwitch/1 -> PeakAmp RAM3/1, PeakIndx RAM3/1
  WeSwitch4/1 -> PeakIndx RAM2/3, PeakAmp RAM2/3
  ENSwitch1/1 -> PeakIndx RAM2/4, PeakAmp RAM2/4
  ADDRSwitch1/1 -> PeakIndx RAM2/1, PeakAmp RAM2/1
  Mux18/1 -> EOFDataMAG2/1
  PeakAmp RAM3/1 -> MAGOutSwitch/3  "MAGPeak2"
  PeakIndx RAM3/1 -> INDXOutSwitch/3  "Peakindx2"
  ENSwitch2/1 -> PeakAmp RAM4/4, PeakIndx RAM4/4
  ADDRSwitch2/1 -> PeakAmp RAM4/1, PeakIndx RAM4/1
  WeSwitch3/1 -> PeakIndx RAM1/3, PeakAmp RAM1/3
  ENSwitch3/1 -> PeakIndx RAM1/4, PeakAmp RAM1/4
  ADDRSwitch3/1 -> PeakIndx RAM1/1, PeakAmp RAM1/1
  PeakAmp RAM4/1 -> MAGOutSwitch1/3  "MAGPeak2"
  PeakIndx RAM4/1 -> INDXOutSwitch1/3  "Peakindx2"
  WeSwitch2/1 -> PeakAmp RAM4/3, PeakIndx RAM4/3
  WinReal2/1 -> Convert2/1
  WinImag2/1 -> Convert4/1
  WinImag1/1 -> Convert5/1
  TX1SimQOut/1 -> Complex Multiplier 6.2/2
  TX1SimIOut/1 -> Complex Multiplier 6.2/3
  Complex Multiplier 6.2/2 -> Convert8/1
  Subsystem/2(FFTtlast) -> TlastVel/1
  RX Lowpass Filter/2(dataOUT) -> WinReal1/1, Gateway Out10/1
  RX Lowpass Filter1/1(dataOUT) -> WinImag1/1
  ROM/1 -> WinReal1/2, WinImag1/2, WinReal2/2, WinImag2/2
  Complex Multiplier 6.2/1 -> DC Removal1/3(tready), DC Removal3/3(tready), DC Removal2/3(tready), DC Removal/3(tready)
  FFTTracking/1(FFTIndex) -> Peak Detection1/3(FFTIndexTrack), Peak Detection2/3(FFTIndexTrack)
  Convert3/1 -> Fast Fourier Transform 9.1/4
  Convert5/1 -> Fast Fourier Transform 9.1/3
  FFTTracking/2(PeakSerachEnable) -> Peak Detection1/4(FFTValidMask), Peak Detection2/4(FFTValidMask)
  Peak Detection2/2(DataMag) -> PeakAmp RAM4/2, PeakAmp RAM1/2
  Peak Detection2/5(Tlast_delayed) -> ENSwitch3/3, WeSwitch3/3, ENSwitch2/3, WeSwitch2/3, EOFRAMen1/2, Logical/1, AddrCountPerChirp/1
  Peak Detection2/3(DataINDX) -> PeakIndx RAM1/2, PeakIndx RAM4/2
  Peak Detection2/1(WriteEnable) -> EOFRAMwe1/2
  PreDelayWEDisable/1 -> EOFRAMwe2/1, EOFRAMwe1/1
  Fast Fourier Transform 9.1/3 -> ManualDownsample2/2(IMGin)
  ManualDownsample2/3(OnDataTrig) -> FFTResultRAMSystem/3(WE), FFTTracking/3(DecimatedTrig)
  FFTTracking/3(IQDataADDR) -> FFTResultRAMSystem1/1(AddressA), FFTResultRAMSystem/1(AddressA)
  FFTResultRAMSystem/1(RngRETx1) -> RngReTx1/1
  FFTResultRAMSystem/2(RngIMGTx1) -> RngImagTx1/1
  Subsystem/1(AddrOut) -> FFTResultRAMSystem1/2(AddressB), FFTResultRAMSystem/2(AddressB)
  ReadToggleBool/1 -> ReadENBool1/1
  ReadENBool1/1 -> FFTResultRAMSystem1/5(SwapRAM), FFTResultRAMSystem/5(SwapRAM)
  Fast Fourier Transform 9.2/6 -> ManualDownsample1/1(data_valid), FFTResultRAMSystem1/4(EN)
  Fast Fourier Transform 9.2/4 -> ManualDownsample1/3(REin)
  ManualDownsample1/3(OnDataTrig) -> FFTResultRAMSystem1/3(WE)
  FFTResultRAMSystem1/1(RngRETx1) -> RngReTx2/1
  FFTResultRAMSystem1/2(RngIMGTx1) -> RngImagTx2/1
  Peak Detection1/1(WriteEnable) -> EOFRAMwe2/2
  Peak Detection1/5(Tlast_delayed) -> ENSwitch1/3, WeSwitch4/3, ENSwitch/3, WeSwitch1/3, EOFRAMen3/2
  Peak Detection1/3(DataINDX) -> PeakIndx RAM2/2, PeakIndx RAM3/2
  Peak Detection1/2(DataMag) -> PeakAmp RAM2/2, PeakAmp RAM3/2
  Fast Fourier Transform 9.2/7 -> Peak Detection1/1(Tlast)
  TX2SimQOut/1 -> Complex Multiplier 6.1/2
  Convert4/1 -> Fast Fourier Transform 9.2/3
  Convert2/1 -> Fast Fourier Transform 9.2/4
  ManualDownsample1/1(IMG) -> FFTResultRAMSystem1/7(DataIMG)
  ManualDownsample1/2(RE) -> FFTResultRAMSystem1/6(DataRE)
  Fast Fourier Transform 9.1/4 -> ManualDownsample2/3(REin)
  Complex Multiplier 6.1/2 -> Convert7/1
  Complex Multiplier 6.1/3 -> Convert9/1
  RX Lowpass Filter2/1(dataOUT) -> WinImag2/1
  RX Lowpass Filter3/1(dataOUT) -> WinReal2/1
  Complex Multiplier 6.2/3 -> Convert6/1
  Gateway Out9/1 -> Scope3/1
  Gateway Out10/1 -> Scope3/2
  Gateway Out12/1 -> Scope3/3
  Gateway Out11/1 -> Scope3/4
  WinReal1/1 -> Convert3/1, Gateway Out12/1
  ReadENBool/1 -> FFTResultRAMSystem1/8(TransmitSel), FFTResultRAMSystem/8(TransmitSel), Subsystem/1(tvalid), TreadyVel/1, Counter2/1
  EOChirp/1 -> DC Removal1/2(tlast), DC Removal3/2(tlast), DC Removal2/2(tlast), DC Removal/2(tlast), Fast Fourier Transform 9.1/6, Fast Fourier Transform 9.2/6
  Fast Fourier Transform 9.1/6 -> FFTTracking/2(StatusReady), FFTTracking/1(data_Active), ManualDownsample2/1(data_valid), FFTResultRAMSystem/4(EN)
  TX1_REFQOut/1 -> Delay/1
  TX2_REFQOut/1 -> Delay2/1
  TX2SimIOut/1 -> Complex Multiplier 6.1/3
  Convert/1 -> Complex Multiplier 6.1/6
  Convert1/1 -> Complex Multiplier 6.2/6
  Delay/1 -> CMult1/1
  Delay1/1 -> Convert1/1
  Delay2/1 -> CMult/1
  Delay3/1 -> Convert/1
  AddSub/1 -> Gateway Out11/1, Peak Detection2/2(FFTInput)
  Mult4/1 -> AddSub/2
  ManualDownsample2/5(PassRE) -> Mult4/2, Mult4/1
  Mult5/1 -> AddSub/1
  ManualDownsample2/4(PassIMG) -> Mult5/1, Mult5/2
  RX Lowpass Filter/1(tready) -> WindowPeriod/1, Fast Fourier Transform 9.1/5, Fast Fourier Transform 9.2/5
  Convert6/1 -> Gateway Out9/1, DC Removal/1(DataIN)
  Convert8/1 -> DC Removal1/1(DataIN)
  Convert7/1 -> DC Removal2/1(DataIN)
  Convert9/1 -> DC Removal3/1(DataIN)
  DC Removal/1(DataOUT) -> RX Lowpass Filter/2(dataIN)
  DC Removal/2(treadyOUT) -> RX Lowpass Filter/1(validIN)
  DC Removal1/1(DataOUT) -> RX Lowpass Filter1/1(dataIN)
  DC Removal2/1(DataOUT) -> RX Lowpass Filter2/1(dataIN)
  DC Removal3/1(DataOUT) -> RX Lowpass Filter3/1(dataIN)
  Fast Fourier Transform 9.2/3 -> ManualDownsample1/2(IMGin)
  ManualDownsample1/4(PassIMG) -> Mult7/2, Mult7/1
  ManualDownsample1/5(PassRE) -> Mult6/2, Mult6/1
